simulink model "prob5"  (R2020b)
settings: Solver=VariableStepAuto  StartTime=0.0  StopTime=10  RelTol=1e-3
model workspace (MAT data in the model file):
  C = 1e-05
  R = 10
settings Model: Creator=nadee  LastModifiedBy=nadee

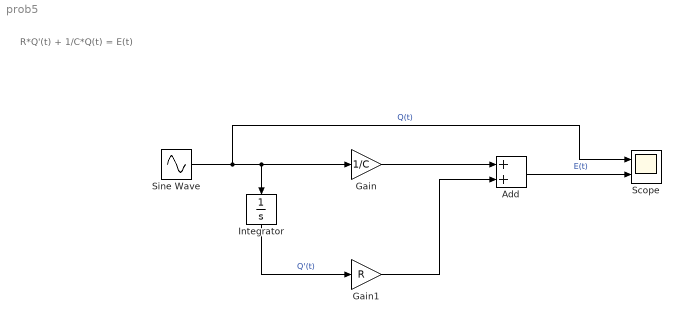
== system prob5 ==
  note: R*Q'(t) + 1/C*Q(t) = E(t)
  Add : Sum
  Gain : Gain  Gain=1/C
  Gain1 : Gain  Gain=R
  Integrator : Integrator
  Scope : Scope  NumInputPorts=2
  Sine Wave : Sin  SampleTime=0
  wires:
  Add/1 -> Scope/2  "E(t)"
  Integrator/1 -> Gain1/1  "Q'(t)"
  Sine Wave/1 -> Scope/1, Integrator/1, Gain/1  "Q(t)"
  Gain1/1 -> Add/2
  Gain/1 -> Add/1
